simulink model "PID"  (R2020a)
settings: Solver=ode3  StartTime=0.0  StopTime=60  FixedStep=0.1  RelTol=1e-3
PostLoadFcn:
  | OPCua_PID([], 'init', true);
  | set_point = [[0 0]; [5 2]; [25 -2]; [35 0]];
  | man_mode = [[0 0]; [40 1]; [50 0]];
  | man_u = [[0 0]; [30 2]];
  | reset = [[0 0]; [35 1]; [36 0]];
InitFcn:
  | V = 5;
  | T1 = 4;
  | T2 = 2;
  | Tsum = 0.5;
  | 
  | TI = 2 * V * Tsum;
  | KP = (T1 + T2) / TI;
  | TD = (T1 * T2)  / TI;
  | OPCua_PID([], 'update', true, 'KP', KP, 'TI', TI, 'TD', TD);
StopFcn:
  | OPCua_PID([], 'reset', true);
libraries: sldrtlib x1
CloseFcn:
  | OPCua_PID([], 'finish', true);
settings Model: Creator=User  LastModifiedBy=User
settings SolverCC: ConcurrentTasks=on
settings DataIOCC: SaveOutput=off  SignalLogging=off  DSMLogging=off  SaveTime=off  ReturnWorkspaceOutputs=off
settings RTWCC: Description=Simulink Desktop Real-Time  SystemTargetFile=sldrt.tlc  TemplateMakefile=sldrt.tmf  RTWCompilerOptimization=on
settings CodeAppCC: MaxIdLength=95
settings SimulinkDesktopRealTimeCC: TargetPreCompLibLocation=C:\Program Files\MATLAB\R2020a\toolbox\sldrt\lib\win64

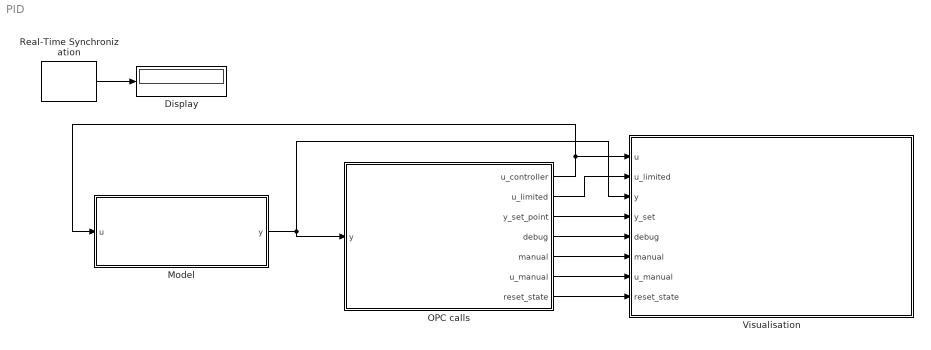
== system PID ==
  Display : Display
  Model : Subsystem  TreatAsAtomicUnit=on
  OPC calls : Subsystem  TreatAsAtomicUnit=on
  Real-Time Synchronization : sldrtlib/Real-Time Synchronization  SampleTime=0.1  MaxMissedTicks=Inf  ShowMissedTicks=on  YieldWhenWaiting=off
  Visualisation : Subsystem  TreatAsAtomicUnit=on
  wires:
  Real-Time Synchronization/1 -> Display/1
  Model/1(y) -> Visualisation/3(y), OPC calls/1(y)
  OPC calls/3(y_set_point) -> Visualisation/4(y_set)
  OPC calls/1(u_controller) -> Model/1(u), Visualisation/1(u)
  OPC calls/2(u_limited) -> Visualisation/2(u_limited)
  OPC calls/4(debug) -> Visualisation/5(debug)
  OPC calls/5(manual) -> Visualisation/6(manual)
  OPC calls/6(u_manual) -> Visualisation/7(u_manual)
  OPC calls/7(reset_state) -> Visualisation/8(reset_state)

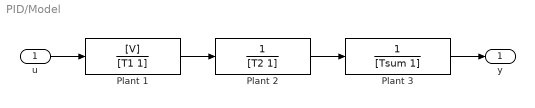
== system PID/Model ==
  u : Inport
  Plant 1 : TransferFcn  Numerator=[V]  Denominator=[T1 1]
  Plant 2 : TransferFcn  Denominator=[T2 1]
  Plant 3 : TransferFcn  Denominator=[Tsum 1]
  y : Outport
  wires:
  Plant 1/1 -> Plant 2/1
  Plant 2/1 -> Plant 3/1
  u/1 -> Plant 1/1
  Plant 3/1 -> y/1

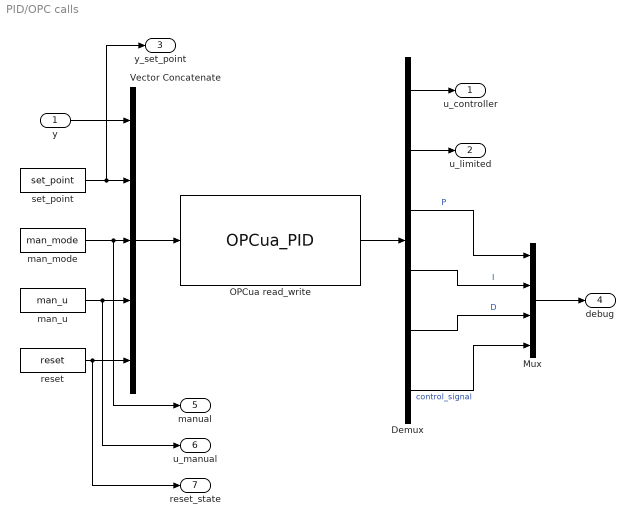
== system PID/OPC calls ==
  y : Inport
  Demux : Demux  Outputs=6
  Mux : Mux
  OPCua read_write : MATLABFcn  MATLABFcn=OPCua_PID  OutputDimensions=6
  Vector Concatenate : Concatenate  NumInputs=5
  man_mode : FromWorkspace  VariableName=man_mode  SampleTime=-1  Interpolate=off  OutputAfterFinalValue=Holding final value
  man_u : FromWorkspace  VariableName=man_u  SampleTime=-1  Interpolate=off  OutputAfterFinalValue=Holding final value
  reset : FromWorkspace  VariableName=reset  SampleTime=-1  Interpolate=off  OutputAfterFinalValue=Holding final value
  set_point : FromWorkspace  VariableName=set_point  SampleTime=-1  Interpolate=off  OutputAfterFinalValue=Holding final value
  u_controller : Outport
  u_limited : Outport  Port=2
  y_set_point : Outport  Port=3
  debug : Outport  Port=4
  manual : Outport  Port=5
  u_manual : Outport  Port=6
  reset_state : Outport  Port=7
  wires:
  Vector Concatenate/1 -> OPCua read_write/1
  OPCua read_write/1 -> Demux/1
  Demux/1 -> u_controller/1
  Demux/2 -> u_limited/1
  set_point/1 -> y_set_point/1, Vector Concatenate/2
  y/1 -> Vector Concatenate/1
  man_mode/1 -> manual/1, Vector Concatenate/3
  Demux/4 -> Mux/2  "I"
  Demux/5 -> Mux/3  "D"
  Demux/6 -> Mux/4  "control_signal"
  Mux/1 -> debug/1
  Demux/3 -> Mux/1  "P"
  reset/1 -> reset_state/1, Vector Concatenate/5
  man_u/1 -> u_manual/1, Vector Concatenate/4

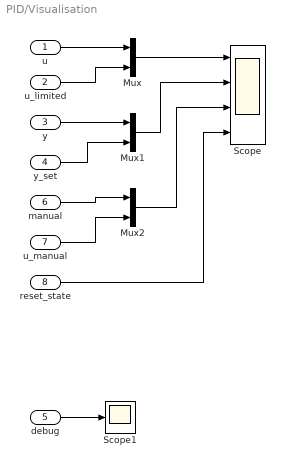
== system PID/Visualisation ==
  u : Inport
  u_limited : Inport  Port=2
  y : Inport  Port=3
  y_set : Inport  Port=4
  debug : Inport  Port=5
  manual : Inport  Port=6
  u_manual : Inport  Port=7
  reset_state : Inport  Port=8
  Mux : Mux  Inputs=2
  Mux1 : Mux  Inputs=2
  Mux2 : Mux  Inputs=2
  Scope : Scope  NumInputPorts=4
  Scope1 : Scope
  wires:
  Mux/1 -> Scope/1
  u/1 -> Mux/1
  u_limited/1 -> Mux/2
  y/1 -> Mux1/1
  y_set/1 -> Mux1/2
  Mux1/1 -> Scope/2
  debug/1 -> Scope1/1
  manual/1 -> Mux2/1
  u_manual/1 -> Mux2/2
  Mux2/1 -> Scope/3
  reset_state/1 -> Scope/4
